simulink model "sccc_sim"  (Simulink 6.0)
settings: Solver=ode45  SolverMode=SingleTasking  StartTime=0.0  StopTime=500  RelTol=1e-3
PostLoadFcn:
  | sccc_setup;
undefined symbols (not defined in the file or in its folder): Max, SCCC_len, SCCC_numIter, SCCC_Var, slcm
libraries: commcnvcod2 x4, commblkintrlv2 x3, dspsrcs4 x2, commchan2 x1, commrandsrc2 x1, dspsigops x1, dspbuff3 x1, commsink2 x1, dspsigattribs x1, dspstat3 x1, commutil2 x1
CloseFcn:
  | clear SCCC_EbN0dB SCCC_R SCCC_Var SCCC_len SCCC_numIter SCCC_seed SCCC_trellis1 SCCC_trellis2 scccSigsOut
settings Model: CovMetricSettings=d  Creator=kkwong  LastModifiedBy=akansal  ExtModeAutoUpdateStatusClock=off
settings SolverCC: ZeroCrossControl=DisableAll
settings DataIOCC: LimitDataPoints=off  SaveOutput=off  SaveTime=off  SignalLoggingName=scccSigsOut
settings OptimizationCC: BlockReduction=off  BooleanDataType=off  InlineParams=on
settings DebuggingCC: CheckExecutionContextPreStartOutputMsg=on  CheckExecutionContextRuntimeOutputMsg=on  SolverPrmCheckMsg=none
settings HardwareCC: TargetUnknown=on
settings CodeAppCC: IgnoreCustomStorageClasses=off
settings SFSimCC: SFSimApplyToAllLibs=on  SFSimBuildMode=Incremental

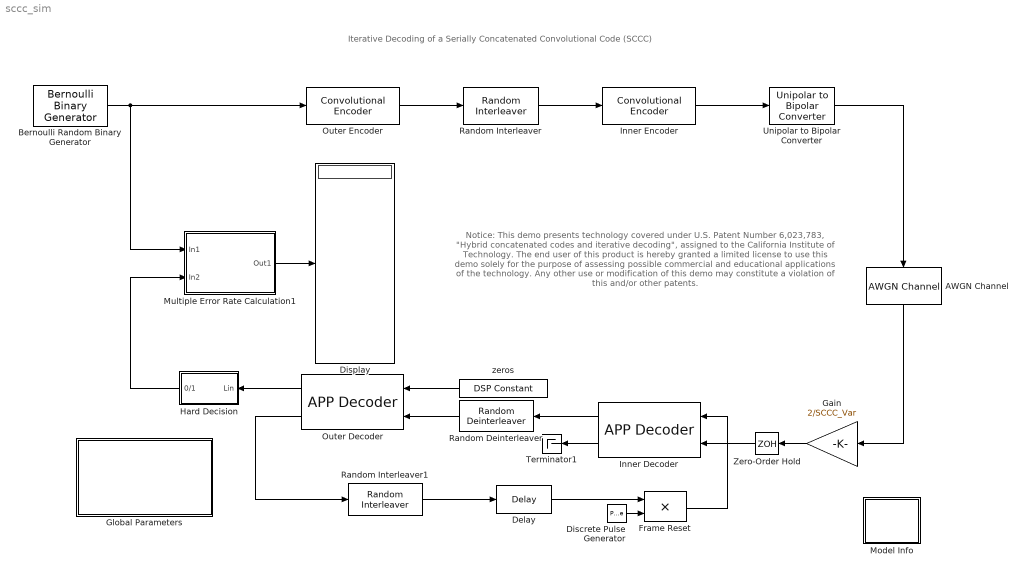
== system sccc_sim ==
  note: Notice: This demo presents technology
      | covered under U.S. Patent Number 6,023,783,
      | "Hybrid concatenated codes and iterative decoding",
      | assigned to the California Institute of Technology.
      |
      | The end user of this product is hereby granted a limited license
      | to use this demo solely for the purpose of  assessing
      | possible commercial and educational applications of the
      | technology. Any other use or modification of this demo
      | may constitute a violation of this and/or other patents.
  note: Iterative Decoding of a Serially Concatenated Convolutional Code (SCCC)
  AWGN Channel : commchan2/AWGN Channel  Orientation=down  seed=123449  noiseMode=Variance from mask  EbNodB=10  EsNodB=0  SNRdB=10  bitsPerSym=1  Ps=1  Tsym=1/len/3  variance=SCCC_Var
  Bernoulli Random Binary Generator : commrandsrc2/Bernoulli Binary Generator  P=0.5  seed=12343  Ts=SCCC_numIter/SCCC_len  frameBased=on  sampPerFrame=SCCC_len  orient=off
  Delay : dspsigops/Delay  dly_unit=Samples  delay=SCCC_len*2  ic_detail=off  dif_ic_for_ch=off  dif_ic_for_dly=off  ic=0  reset_popup=None
  Discrete Pulse Generator : DiscretePulseGenerator  Period=SCCC_numIter  PulseWidth=SCCC_numIter-1  PhaseDelay=1
  Display : Display
      settings: Format=short_e
  Frame Reset : Product  SaturateOnIntegerOverflow=on  InputSameDT=on
  Gain : Gain  Orientation=left  Gain=2/SCCC_Var  SaturateOnIntegerOverflow=on
  Global Parameters : Subsystem  PropExecContextAcrossSSBoundary=on  mask(Global Parameters){SCCC_EbN0dB=1.5, SCCC_len=1024, SCCC_numIter=6, SCCC_seed=19046}
      mask prompts: SCCC_EbN0dB "Eb/No:"; SCCC_len "Block size:"; SCCC_numIter "Number of iterations:"; SCCC_seed "Seed:"
      mask help: Load global parameters in MATLAB workspace.
      mask init:
      | sccc_setup;
      mask CallbackString: sccc_setup|sccc_setup|sccc_setup|sccc_setup
      mask Display:
      | disp(['Eb/No   ' num2str(SCCC_EbN0dB,'%3.1f') 'dB'
      | sprintf('\n') 'Block size   ' num2str(SCCC_len,'%7.0f')
      | sprintf('\n') 'Iterations   ' num2str(SCCC_numIter,'%3.0f')
      | sprintf('\n') 'Seed   ' num2str(SCCC_seed,'%7.0f')])
  Hard Decision : Subsystem  Orientation=left  PropExecContextAcrossSSBoundary=on
      mask Type: Hard Decision
      mask Description: Likelihood to binary transformation.
  Inner Decoder : commcnvcod2/APP Decoder  Orientation=left  trellis=poly2trellis([3 3],[7 0 5;0 7 6],[7 7])  termMethod=Truncated  algorithm=Max*  maxStarNumScaleBits=3
  Inner Encoder : commcnvcod2/Convolutional Encoder  trellis=poly2trellis([3 3],[7 0 5;0 7 6],[7 7])  reset=On each frame
  Model Info : Subsystem  LoadFcn=slcm LoadBlock;  InitFcn=slcm('UpdateAllCMBlocksInThisModelInit')  PropExecContextAcrossSSBoundary=on  mask(CMBlock){InitialSaveTempField=, InitialBlockCM=none, BlockCM=none, Frame=on, SaveTempField=, DisplayStringWithTags=Info, MaskDisplayString=Info, HorizontalTextAlignment=Center, LeftAlignmentValue=0.5, SourceBlockDiagram=sccc_sim, TagMaxNumber=20, CMTag1=, CMTag2=, CMTag3=, CMTag4=, CMTag5=, CMTag6=, CMTag7=, CMTag8=, CMTag9=, CMTag10=, CMTag11=, CMTag12=, CMTag13=, CMTag14=, CMTag15=, CMTag16=, CMTag17=, CMTag18=, CMTag19=, CMTag20=}
      mask help: This block allows revision control information to be displayed within the model.
      settings: CopyFcn=slcm CopyBlock;  DeleteFcn=slcm Cancel;  PostSaveFcn=slcm('UpdateAllCMBlocksInThisModel')  NameChangeFcn=slcm Rename;  OpenFcn=commdemohelp;
      mask Display: text(str2num(LeftAlignmentValue), 0.5, MaskDisplayString, 'HorizontalAlignment', HorizontalTextAlignment)
  Multiple Error Rate Calculation1 : Subsystem  PropExecContextAcrossSSBoundary=on
      mask Display: disp('Multiple\nIteration\nError Rate\nCalculation')
  Outer Decoder : commcnvcod2/APP Decoder  Orientation=left  trellis=poly2trellis(3, [7 5],7)  termMethod=Truncated  algorithm=Max*  maxStarNumScaleBits=3
  Outer Encoder : commcnvcod2/Convolutional Encoder  trellis=poly2trellis(3, [7 5],7)  reset=On each frame
  Random Deinterleaver : commblkintrlv2/Random Deinterleaver  Orientation=left  N=SCCC_len*2  seed=SCCC_seed
  Random Interleaver : commblkintrlv2/Random Interleaver  N=SCCC_len*2  seed=SCCC_seed
  Random Interleaver1 : commblkintrlv2/Random Interleaver  N=SCCC_len*2  seed=SCCC_seed
  Terminator1 : Terminator
  Unipolar to Bipolar Converter : commutil2/Unipolar to Bipolar Converter  M=2  polarity=Positive
  Zero-Order Hold : ZeroOrderHold  Orientation=left  SampleTime=SCCC_numIter
  zeros : dspsrcs4/DSP Constant  Orientation=left  Value=zeros(SCCC_len,1)  SampleMode=Discrete  discreteOutput=Frame-based  continuousOutput=Sample-based  sampTime=1  framePeriod=1  dataType=Inherit from 'Constant value'  isSigned=on  wordLen=16  udDataType=sfix(16)  fracBitsMode=Best precision  numFracBits=15  InterpretAs1D=off  Ts=1  FramebasedOutput=on
  wires:
  AWGN Channel/1 -> Gain/1
  Unipolar to Bipolar Converter/1 -> AWGN Channel/1
  Bernoulli Random Binary Generator/1 -> Multiple Error Rate Calculation1/1(In1), Outer Encoder/1
  Outer Encoder/1 -> Random Interleaver/1
  Random Interleaver/1 -> Inner Encoder/1
  Inner Encoder/1 -> Unipolar to Bipolar Converter/1
  Inner Decoder/2 -> Terminator1/1
  Inner Decoder/1 -> Random Deinterleaver/1
  Random Deinterleaver/1 -> Outer Decoder/2
  Outer Decoder/2 -> Random Interleaver1/1
  zeros/1 -> Outer Decoder/1
  Frame Reset/1 -> Inner Decoder/1
  Random Interleaver1/1 -> Delay/1
  Outer Decoder/1 -> Hard Decision/1(Lin)
  Hard Decision/1(0/1) -> Multiple Error Rate Calculation1/2(In2)
  Multiple Error Rate Calculation1/1(Out1) -> Display/1
  Gain/1 -> Zero-Order Hold/1
  Discrete Pulse Generator/1 -> Frame Reset/2
  Delay/1 -> Frame Reset/1
  Zero-Order Hold/1 -> Inner Decoder/2

== system sccc_sim/Global Parameters ==

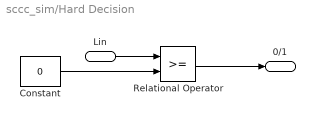
== system sccc_sim/Hard Decision ==
  Lin : Inport  LatchInput=off
  Constant : Constant  Value=0
  Relational Operator : RelationalOperator  InputSameDT=on
  0/1 : Outport
  wires:
  Relational Operator/1 -> 0/1/1
  Lin/1 -> Relational Operator/1
  Constant/1 -> Relational Operator/2

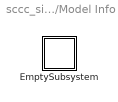
== system sccc_sim/Model Info ==
  EmptySubsystem : Subsystem  PropExecContextAcrossSSBoundary=on

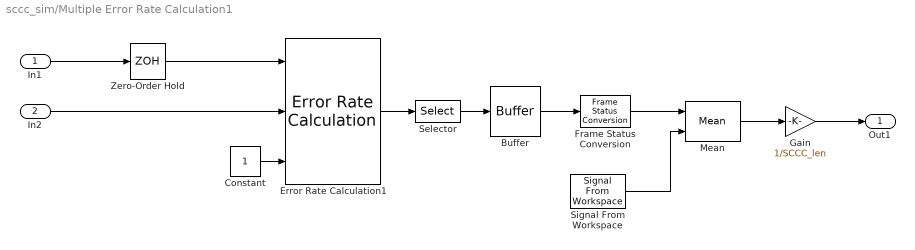
== system sccc_sim/Multiple Error Rate Calculation1 ==
  In1 : Inport  LatchInput=off
  In2 : Inport  Port=2  LatchInput=off
  Buffer : dspbuff3/Buffer  N=SCCC_numIter  V=0  ic=0
  Constant : Constant
  Error Rate Calculation1 : commsink2/Error Rate Calculation  N=0  st_delay=0  cp_mode=Entire frame  subframe=[]  PMode=Port  WsName=ErrorVec1  RsMode2=on
  Frame Status Conversion : dspsigattribs/Frame Status Conversion  growRefPort=off  outframe=Sample-based
  Gain : Gain  Gain=1/SCCC_len  SaturateOnIntegerOverflow=on
  Mean : dspstat3/Mean  run=on  reset_popup=Non-zero sample
  Selector : Selector  Elements=2  InputPortWidth=3
  Signal From Workspace : dspsrcs4/Signal From Workspace  X=[1 1]  Ts=SCCC_numIter  nsamps=1  OutputAfterFinalValue=Setting to zero
  Zero-Order Hold : ZeroOrderHold
  Out1 : Outport
  wires:
  In1/1 -> Zero-Order Hold/1
  Error Rate Calculation1/1 -> Selector/1
  Selector/1 -> Buffer/1
  In2/1 -> Error Rate Calculation1/2
  Buffer/1 -> Frame Status Conversion/1
  Frame Status Conversion/1 -> Mean/1
  Zero-Order Hold/1 -> Error Rate Calculation1/1
  Constant/1 -> Error Rate Calculation1/3
  Mean/1 -> Gain/1
  Gain/1 -> Out1/1
  Signal From Workspace/1 -> Mean/2

== system sccc_sim/Model Info/EmptySubsystem ==
